simulink model "model2d"  (R2020a)
settings: Solver=VariableStepAuto  StartTime=0.0  StopTime=10.0  RelTol=1e-3
values from neighbouring files (symbols this model uses):
  a_phi1 = 2.87    [a2p2.m]    (also in p2c.m; p2c_e.m; p2f.m; p2g.m)
  a_phi2 = -0.65    [a2p2.m]    (also in p2c.m; p2c_e.m; p2f.m; p2g.m)
  d = 1.5*pi/180    (= 0.0261799387799)    [a2p2.m]    (also in p2c_e.m)
  g = 9.81    [a2p2.m]    (also in p2c_e.m; p2f.m; p2g.m)
  kd_phi = (2*zeta_phi*omega_n_phi - a_phi1)/a_phi2    [a2p2.m]    (also in p2c.m = 2.24; p2c_e.m; p2f.m; p2g.m)
  ki_chi = (omega_n_chi)^2 * V_g/g    [a2p2.m]    (also in p2c_e.m; p2f.m; p2g.m)
  kp_chi = 2*zeta_chi*omega_n_chi*V_g/g    [a2p2.m]    (also in p2c_e.m; p2f.m; p2g.m)
  kp_phi = (delta_max_a/e_max_a)*sign(a_phi2)    [a2p2.m]    (also in p2c.m = delta_max / e_phimax * sign(a_phi2); p2c_e.m; p2f.m; p2g.m)
  V_g = V_a    (= 580)    [a2p2.m]    (also in p2c_e.m; p2f.m; p2g.m)
libraries: simulink_extras x3
settings Model: Creator=ivermyklebust  LastModifiedBy=ivermyklebust

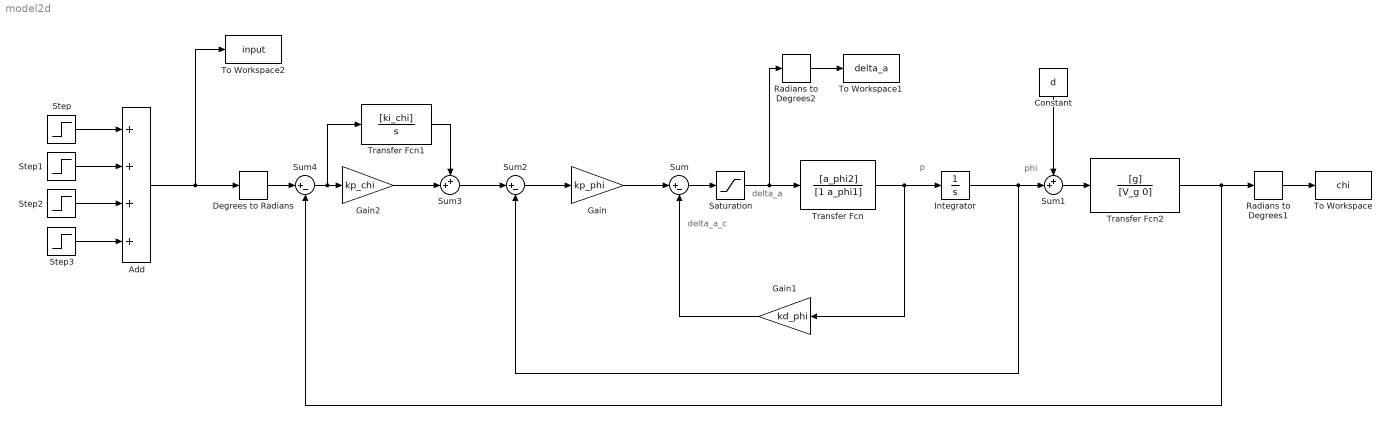
== system model2d ==
  note: phi
  note: p
  note: delta_a
  note: delta_a_c
  Add : Sum  Inputs=++++
  Constant : Constant  Value=d
  Degrees to Radians : simulink_extras/Transformations/Degrees to Radians
  Gain : Gain  Gain=kp_phi
  Gain1 : Gain  Gain=kd_phi
  Gain2 : Gain  Gain=kp_chi
  Integrator : Integrator
  Radians to Degrees1 : simulink_extras/Transformations/Radians to Degrees
  Radians to Degrees2 : simulink_extras/Transformations/Radians to Degrees
  Saturation : Saturate  UpperLimit=pi/6  LowerLimit=-pi/6
  Step : Step  Time=100  After=7.5  SampleTime=0
  Step1 : Step  Time=150  After=7.5  SampleTime=0
  Step2 : Step  Time=250  After=-7.5  SampleTime=0
  Step3 : Step  Time=300  After=0  SampleTime=0
  Sum : Sum  Inputs=|+-
  Sum1 : Sum  Inputs=++|
  Sum2 : Sum  Inputs=|+-
  Sum3 : Sum  Inputs=++|
  Sum4 : Sum  Inputs=|+-
  To Workspace : ToWorkspace  VariableName=chi  SaveFormat=Timeseries  SampleTime=-1
  To Workspace1 : ToWorkspace  VariableName=delta_a  SaveFormat=Timeseries  SampleTime=-1
  To Workspace2 : ToWorkspace  VariableName=input  SaveFormat=Timeseries  SampleTime=-1
  Transfer Fcn : TransferFcn  Numerator=[a_phi2]  Denominator=[1 a_phi1]
  Transfer Fcn1 : TransferFcn  Numerator=[ki_chi]  Denominator=[1 0]
  Transfer Fcn2 : TransferFcn  Numerator=[g]  Denominator=[V_g 0]
  wires:
  Gain/1 -> Sum/1
  Saturation/1 -> Radians to Degrees2/1, Transfer Fcn/1
  Transfer Fcn/1 -> Gain1/1, Integrator/1
  Gain1/1 -> Sum/2
  Sum/1 -> Saturation/1
  Constant/1 -> Sum1/1
  Sum2/1 -> Gain/1
  Sum1/1 -> Transfer Fcn2/1
  Integrator/1 -> Sum2/2, Sum1/2
  Sum3/1 -> Sum2/1
  Transfer Fcn1/1 -> Sum3/1
  Gain2/1 -> Sum3/2
  Sum4/1 -> Transfer Fcn1/1, Gain2/1
  Transfer Fcn2/1 -> Sum4/2, Radians to Degrees1/1
  Radians to Degrees1/1 -> To Workspace/1
  Add/1 -> To Workspace2/1, Degrees to Radians/1
  Degrees to Radians/1 -> Sum4/1
  Step/1 -> Add/1
  Step3/1 -> Add/4
  Step2/1 -> Add/3
  Step1/1 -> Add/2
  Radians to Degrees2/1 -> To Workspace1/1
